simulink library "SUB_ECU_CruiseController"  (R2018a)
settings: Solver=VariableStepAuto  StartTime=0.0  StopTime=10.0  RelTol=1e-3
undefined symbols (not defined in the file or in its folder): ENUM_J1939_SWITCH_T
libraries: PTC_MBDS_LIB x17, simulink x4, simulink_extras x1
settings Model: Creator=Sundeep.Tuteja  LastModifiedBy=Sundeep.Tuteja

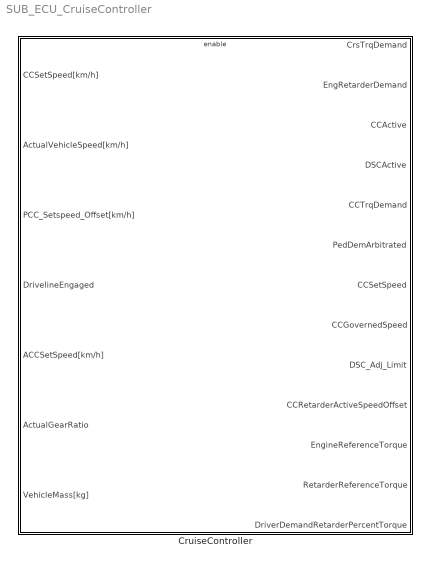
== system SUB_ECU_CruiseController ==
  CruiseController : Subsystem

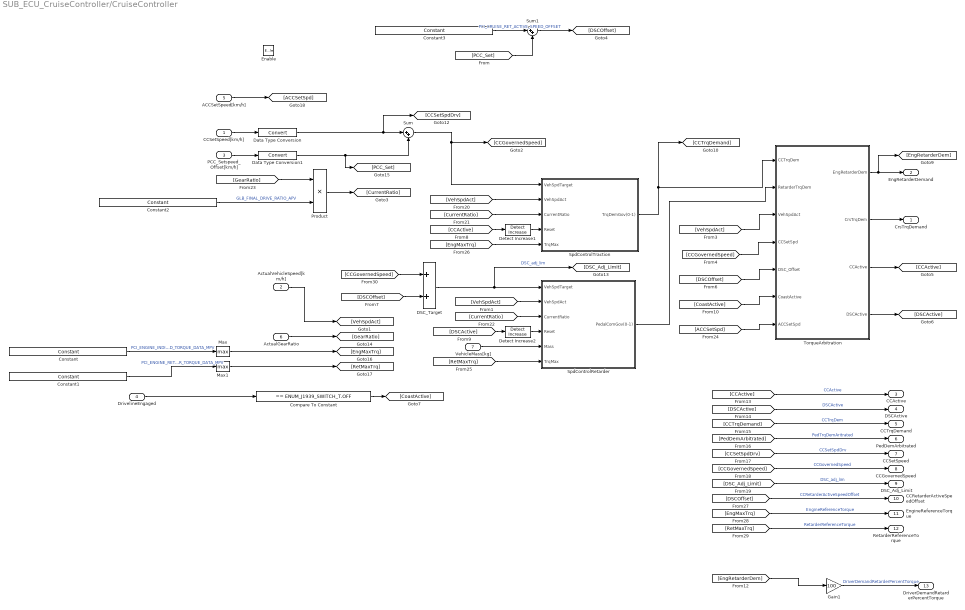
== system SUB_ECU_CruiseController/CruiseController ==
  CCSetSpeed[km/h] : Inport  Unit=km/h
  ActualVehicleSpeed[km/h] : Inport  Port=2  Unit=km/h
  PCC_Setspeed_Offset[km/h] : Inport  Port=3  Unit=km/h
  DrivelineEngaged : Inport  Port=4
  ACCSetSpeed[km/h] : Inport  Port=5  Unit=km/h
  ActualGearRatio : Inport  Port=6
  VehicleMass[kg] : Inport  Port=7  Unit=kg
  Enable : EnablePort
  Compare To Constant : simulink/Logic and Bit Operations/Compare To Constant  relop===  const=ENUM_J1939_SWITCH_T.OFF  OutDataTypeStr=boolean
  Constant : PTC_MBDS_LIB/Extras/Sources/Constant  Value2=PCI_ENGINE_INDICATED_TORQUE_DATA_MPV  PTC_MBDS_BlockVersion=5.41  PTC_BlockType=PTC_MBDS_Constant
      settings: SourceProductName=PACCAR Technical Center MBDS Library
      settings: AttributesFormatString=|
      | Value: <1 X 16>
      | Unit: 'N*m'
  Constant1 : PTC_MBDS_LIB/Extras/Sources/Constant  Value2=PCI_ENGINE_RETARDER_TORQUE_DATA_MPV  PTC_MBDS_BlockVersion=5.41  PTC_BlockType=PTC_MBDS_Constant
      settings: SourceProductName=PACCAR Technical Center MBDS Library
      settings: AttributesFormatString=|
      | Value: <1 X 16>
      | Unit: 'N*m'
  Constant2 : PTC_MBDS_LIB/Extras/Sources/Constant  Value2=GLB_FINAL_DRIVE_RATIO_APV  PTC_MBDS_BlockVersion=5.41  PTC_BlockType=PTC_MBDS_Constant
      settings: SourceProductName=PACCAR Technical Center MBDS Library
      settings: AttributesFormatString=|
      | Value: 2.64
      | Unit: '1'
  Constant3 : PTC_MBDS_LIB/Extras/Sources/Constant  Value2=PCI_CRUISE_RET_ACTIVE_SPEED_OFFSET  PTC_MBDS_BlockVersion=5.41  PTC_BlockType=PTC_MBDS_Constant
      settings: SourceProductName=PACCAR Technical Center MBDS Library
      settings: AttributesFormatString=|
      | Value: 4.5
      | Unit: 'km/h'
  DSC_Target : Sum
  Data Type Conversion : DataTypeConversion  SaturateOnIntegerOverflow=on
  Data Type Conversion1 : DataTypeConversion  SaturateOnIntegerOverflow=on
  Detect Increase1 : simulink/Logic and Bit Operations/Detect Increase  RequirementInfo={} %GIDa_b76eb822_ce3a_4747_9d7e_f46469754665  vinit=0.0  OutDataTypeStr=boolean
  Detect Increase2 : simulink/Logic and Bit Operations/Detect Increase  RequirementInfo={} %GIDa_136ab55b_ef96_43b5_a251_f5d87d11e975  vinit=0.0  OutDataTypeStr=boolean
  Gain1 : Gain  Gain=100
  Max : MinMax  Function=max  OutDataTypeStr=Inherit: Inherit via back propagation  SaturateOnIntegerOverflow=on  InputSameDT=on
  Max1 : MinMax  Function=max  OutDataTypeStr=Inherit: Inherit via back propagation  SaturateOnIntegerOverflow=on  InputSameDT=on
  Product : Product
  SpdControlRetarder : Subsystem
  SpdControlTraction : Subsystem
  Sum : Sum  Inputs=|++
  Sum1 : Sum  Inputs=|++
  TorqueArbitration : Subsystem
  CrsTrqDemand : Outport
  EngRetarderDemand : Outport  Port=2
  CCActive : Outport  Port=3
  DSCActive : Outport  Port=4
  CCTrqDemand : Outport  Port=5
  PedDemArbitrated : Outport  Port=6
  CCSetSpeed : Outport  Port=7
  CCGovernedSpeed : Outport  Port=8
  DSC_Adj_Limit : Outport  Port=9
  CCRetarderActiveSpeedOffset : Outport  Port=10
  EngineReferenceTorque : Outport  Port=11
  RetarderReferenceTorque : Outport  Port=12
  DriverDemandRetarderPercentTorque : Outport  Port=13
  wires:
  CCSetSpeed[km/h]/1 -> Data Type Conversion/1
  DSC_Target/1 -> [DSC_Adj_Limit], SpdControlRetarder/1(VehSpdTarget)  "DSC_adj_lim"
  Constant3/1 -> Sum1/1  "PCI_CRUISE_RET_ACTIVE_SPEED_OFFSET"
  SpdControlRetarder/1(PedalComGov(0-1)) -> TorqueArbitration/2(RetarderTrqDem)
  [VehSpdAct] -> SpdControlRetarder/2(VehSpdAct)
  [VehSpdAct] -> TorqueArbitration/3(VehSpdAct)
  [CCGovernedSpeed] -> DSC_Target/1
  [CCGovernedSpeed] -> TorqueArbitration/4(CCSetSpd)
  [DSCOffset] -> TorqueArbitration/5(DSC_Offset)
  [DSCOffset] -> DSC_Target/2
  TorqueArbitration/2(CrsTrqDem) -> CrsTrqDemand/1
  TorqueArbitration/1(EngRetarderDem) -> [EngRetarderDem], EngRetarderDemand/1
  TorqueArbitration/3(CCActive) -> [CCActive]
  TorqueArbitration/4(DSCActive) -> [DSCActive]
  Detect Increase1/1 -> SpdControlTraction/4(Reset)
  Detect Increase2/1 -> SpdControlRetarder/4(Reset)
  [CCActive] -> Detect Increase1/1
  [DSCActive] -> Detect Increase2/1
  DrivelineEngaged/1 -> Compare To Constant/1
  [CoastActive] -> TorqueArbitration/6(CoastActive)
  [CCActive] -> CCActive/1  "CCActive"
  [DSCActive] -> DSCActive/1  "DSCActive"
  SpdControlTraction/1(TrqDemGov(0-1)) -> TorqueArbitration/1(CCTrqDem), [CCTrqDemand]
  [CCTrqDemand] -> CCTrqDemand/1  "CCTrqDem"
  [PedDemArbitrated] -> PedDemArbitrated/1  "PedTrqDemAritrated"
  Sum/1 -> SpdControlTraction/1(VehSpdTarget), [CCGovernedSpeed]
  PCC_Setspeed_Offset[km/h]/1 -> Data Type Conversion1/1
  [CCSetSpdDrv] -> CCSetSpeed/1  "CCSetSpdDrv"
  [CCGovernedSpeed] -> CCGovernedSpeed/1  "CCGovernedSpeed"
  [DSC_Adj_Limit] -> DSC_Adj_Limit/1  "DSC_adj_lim"
  Constant2/1 -> Product/2  "GLB_FINAL_DRIVE_RATIO_APV"
  ActualVehicleSpeed[km/h]/1 -> [VehSpdAct]
  Product/1 -> [CurrentRatio]
  [VehSpdAct] -> SpdControlTraction/2(VehSpdAct)
  [CurrentRatio] -> SpdControlTraction/3(CurrentRatio)
  [CurrentRatio] -> SpdControlRetarder/3(CurrentRatio)
  VehicleMass[kg]/1 -> SpdControlRetarder/5(Mass)
  ActualGearRatio/1 -> [GearRatio]
  [GearRatio] -> Product/1
  Constant/1 -> Max/1  "PCI_ENGINE_INDICATED_TORQUE_DATA_MPV"
  Max1/1 -> [RetMaxTrq]
  [RetMaxTrq] -> SpdControlRetarder/6(TrqMax)
  [EngMaxTrq] -> SpdControlTraction/5(TrqMax)
  ACCSetSpeed[km/h]/1 -> [ACCSetSpd]
  [ACCSetSpd] -> TorqueArbitration/7(ACCSetSpd)
  Sum1/1 -> [DSCOffset]
  [PCC_Set] -> Sum1/2
  Max/1 -> [EngMaxTrq]
  Constant1/1 -> Max1/1  "PCI_ENGINE_RETARDER_TORQUE_DATA_MPV"
  Compare To Constant/1 -> [CoastActive]
  [DSCOffset] -> CCRetarderActiveSpeedOffset/1  "CCRetarderActiveSpeedOffset"
  [EngMaxTrq] -> EngineReferenceTorque/1  "EngineReferenceTorque"
  [RetMaxTrq] -> RetarderReferenceTorque/1  "RetarderReferenceTorque"
  Data Type Conversion/1 -> [CCSetSpdDrv], Sum/1
  Data Type Conversion1/1 -> [PCC_Set], Sum/2
  Gain1/1 -> DriverDemandRetarderPercentTorque/1  "DriverDemandRetarderPercentTorque"
  [EngRetarderDem] -> Gain1/1

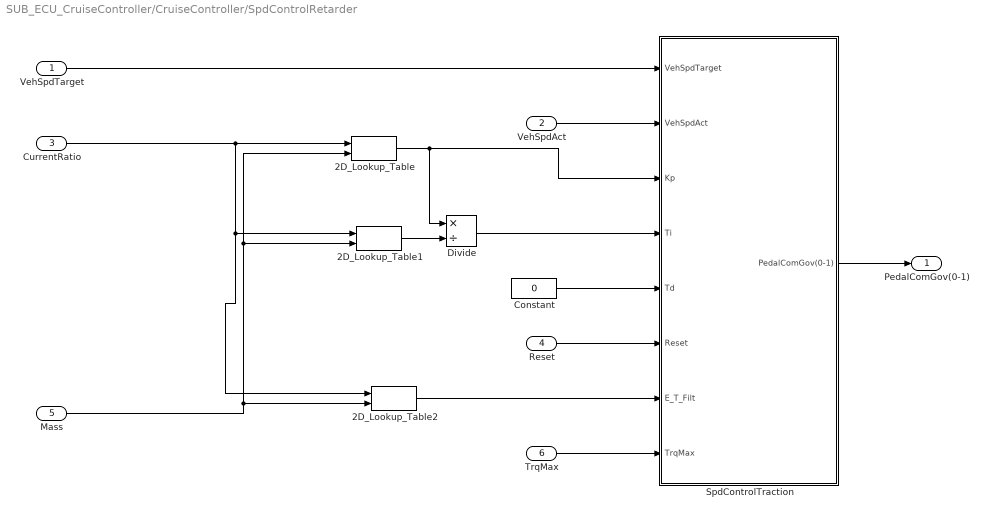
== system SUB_ECU_CruiseController/CruiseController/SpdControlRetarder ==
  VehSpdTarget : Inport
  VehSpdAct : Inport  Port=2
  CurrentRatio : Inport  Port=3
  Reset : Inport  Port=4
  Mass : Inport  Port=5
  TrqMax : Inport  Port=6
  2D_Lookup_Table : PTC_MBDS_LIB/Extras/Lookup Tables/2D_Lookup_Table  ParameterObjectName=PCI_CRUISE_DSC_KP_DATA_MPV  PTC_MBDS_BlockVersion=5.41  PTC_BlockType=PTC_MBDS_2D_Lookup_Table
      settings: SourceProductName=PACCAR Technical Center MBDS Library
      settings: AttributesFormatString=|
      | Row Axis: PCI_CRUISE_DSC_DRIVE_RATIO_MPV ()
      | Column Axis: PCI_CRUISE_DSC_MASS_MPV (kg)
      | Data Axis: PCI_CRUISE_DSC_KP_DATA_MPV ()
  2D_Lookup_Table1 : PTC_MBDS_LIB/Extras/Lookup Tables/2D_Lookup_Table  ParameterObjectName=PCI_CRUISE_DSC_KI_DATA_MPV  PTC_MBDS_BlockVersion=5.41  PTC_BlockType=PTC_MBDS_2D_Lookup_Table
      settings: SourceProductName=PACCAR Technical Center MBDS Library
      settings: AttributesFormatString=|
      | Row Axis: PCI_CRUISE_DSC_DRIVE_RATIO_MPV ()
      | Column Axis: PCI_CRUISE_DSC_MASS_MPV (kg)
      | Data Axis: PCI_CRUISE_DSC_KI_DATA_MPV (1/s)
  2D_Lookup_Table2 : PTC_MBDS_LIB/Extras/Lookup Tables/2D_Lookup_Table  ParameterObjectName=PCI_CRUISE_DSC_ERROR_FILT_T_MPV  PTC_MBDS_BlockVersion=5.41  PTC_BlockType=PTC_MBDS_2D_Lookup_Table
      settings: SourceProductName=PACCAR Technical Center MBDS Library
      settings: AttributesFormatString=|
      | Row Axis: PCI_CRUISE_DSC_DRIVE_RATIO_MPV ()
      | Column Axis: PCI_CRUISE_DSC_MASS_MPV (kg)
      | Data Axis: PCI_CRUISE_DSC_ERROR_FILT_T_MPV (s)
  Constant : Constant  Value=0
  Divide : Product  Inputs=*/
  SpdControlTraction : Subsystem
  PedalComGov(0-1) : Outport
  wires:
  Mass/1 -> 2D_Lookup_Table2/2, 2D_Lookup_Table1/2, 2D_Lookup_Table/2
  VehSpdTarget/1 -> SpdControlTraction/1(VehSpdTarget)
  VehSpdAct/1 -> SpdControlTraction/2(VehSpdAct)
  SpdControlTraction/1(PedalComGov(0-1)) -> PedalComGov(0-1)/1
  Reset/1 -> SpdControlTraction/6(Reset)
  CurrentRatio/1 -> 2D_Lookup_Table/1, 2D_Lookup_Table2/1, 2D_Lookup_Table1/1
  2D_Lookup_Table2/1 -> SpdControlTraction/7(E_T_Filt)
  Constant/1 -> SpdControlTraction/5(Td)
  2D_Lookup_Table/1 -> SpdControlTraction/3(Kp), Divide/1
  2D_Lookup_Table1/1 -> Divide/2
  Divide/1 -> SpdControlTraction/4(Ti)
  TrqMax/1 -> SpdControlTraction/8(TrqMax)

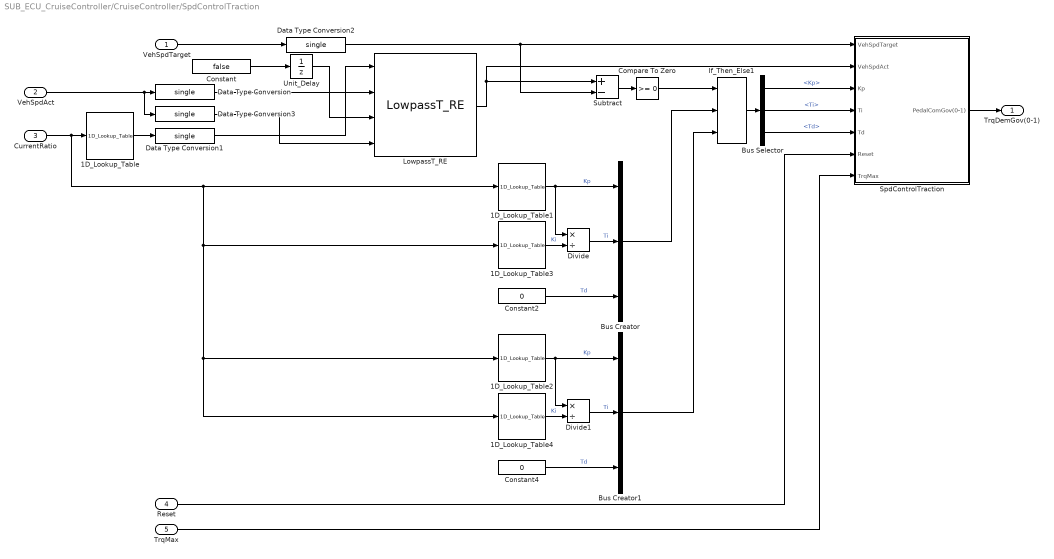
== system SUB_ECU_CruiseController/CruiseController/SpdControlTraction ==
  VehSpdTarget : Inport
  VehSpdAct : Inport  Port=2
  CurrentRatio : Inport  Port=3
  Reset : Inport  Port=4
  TrqMax : Inport  Port=5
  1D_Lookup_Table : PTC_MBDS_LIB/Extras/Lookup Tables/1D_Lookup_Table  ParameterObjectName=PCI_VSPD_FILT_T_DATA_MPV  PTC_MBDS_BlockVersion=5.41  PTC_BlockType=PTC_MBDS_1D_Lookup_Table
      settings: SourceProductName=PACCAR Technical Center MBDS Library
      settings: AttributesFormatString=|
      | X Axis: PCI_DRIVE_RATIO_MPV (1)
      | Y Axis: PCI_VSPD_FILT_T_DATA_MPV (s)
  1D_Lookup_Table1 : PTC_MBDS_LIB/Extras/Lookup Tables/1D_Lookup_Table  ParameterObjectName=PCI_CRUISE_KP_HIGH_MPV  PTC_MBDS_BlockVersion=5.41  PTC_BlockType=PTC_MBDS_1D_Lookup_Table
      settings: SourceProductName=PACCAR Technical Center MBDS Library
      settings: AttributesFormatString=|
      | X Axis: PCI_DRIVE_RATIO_MPV (1)
      | Y Axis: PCI_CRUISE_KP_HIGH_MPV (1)
  1D_Lookup_Table2 : PTC_MBDS_LIB/Extras/Lookup Tables/1D_Lookup_Table  ParameterObjectName=PCI_CRUISE_KP_LOW_MPV  PTC_MBDS_BlockVersion=5.41  PTC_BlockType=PTC_MBDS_1D_Lookup_Table
      settings: SourceProductName=PACCAR Technical Center MBDS Library
      settings: AttributesFormatString=|
      | X Axis: PCI_DRIVE_RATIO_MPV (1)
      | Y Axis: PCI_CRUISE_KP_LOW_MPV ()
  1D_Lookup_Table3 : PTC_MBDS_LIB/Extras/Lookup Tables/1D_Lookup_Table  ParameterObjectName=PCI_CRUISE_KI_HIGH_MPV  PTC_MBDS_BlockVersion=5.41  PTC_BlockType=PTC_MBDS_1D_Lookup_Table
      settings: SourceProductName=PACCAR Technical Center MBDS Library
      settings: AttributesFormatString=|
      | X Axis: PCI_DRIVE_RATIO_MPV (1)
      | Y Axis: PCI_CRUISE_KI_HIGH_MPV (1/s)
  1D_Lookup_Table4 : PTC_MBDS_LIB/Extras/Lookup Tables/1D_Lookup_Table  ParameterObjectName=PCI_CRUISE_KI_LOW_MPV  PTC_MBDS_BlockVersion=5.41  PTC_BlockType=PTC_MBDS_1D_Lookup_Table
      settings: SourceProductName=PACCAR Technical Center MBDS Library
      settings: AttributesFormatString=|
      | X Axis: PCI_DRIVE_RATIO_MPV (1)
      | Y Axis: PCI_CRUISE_KI_LOW_MPV (1/s)
  Bus Creator : BusCreator  Inputs=3
  Bus Creator1 : BusCreator  Inputs=3
  Bus Selector : BusSelector  OutputSignals=Kp,Ti,Td
  Compare To Zero : simulink/Logic and Bit Operations/Compare To Zero  relop=>=  OutDataTypeStr=boolean
  Constant : Constant  Value=false  OutDataTypeStr=boolean
  Constant2 : Constant  Value=0
  Constant4 : Constant  Value=0
  Data Type Conversion{,1..3} (4 alike) : DataTypeConversion  OutDataTypeStr=single
  Divide : Product  Inputs=*/
  Divide1 : Product  Inputs=*/
  If_Then_Else1 : PTC_MBDS_LIB/Extras/Signal Routing/If_Then_Else  PTC_MBDS_BlockVersion=5.41  PTC_BlockType=PTC_MBDS_If_Then_Else
      settings: SourceProductName=PACCAR Technical Center MBDS Library
  LowpassT_RE : PTC_MBDS_LIB/MBDS Standard Library/Extended Operations/Filters/LowpassT_RE  dT_Enabled=off  dT=GLB_FIXED_STEP_SIZE_CPV  E_Enabled=off  R_Enabled=on  IV_Enabled=on  IV=0  PTC_MBDS_BlockVersion=5.41  PTC_BlockType=PTC_MBDS_LowpassT_RE
      settings: AttributesFormatString=dT = %<dT>  SourceProductName=PACCAR Technical Center MBDS Library
  SpdControlTraction : Subsystem
  Subtract : Sum  Inputs=+-
  Unit_Delay : UnitDelay  InitialCondition=true  SampleTime=-1
      settings: AttributesFormatString=Init = %<InitialCondition>
  TrqDemGov(0-1) : Outport
  wires:
  Reset/1 -> SpdControlTraction/6(Reset)
  SpdControlTraction/1(PedalComGov(0-1)) -> TrqDemGov(0-1)/1
  VehSpdTarget/1 -> Data Type Conversion2/1
  CurrentRatio/1 -> 1D_Lookup_Table/1, 1D_Lookup_Table1/1, 1D_Lookup_Table3/1, 1D_Lookup_Table4/1, 1D_Lookup_Table2/1
  VehSpdAct/1 -> Data Type Conversion3/1, Data Type Conversion/1
  Constant/1 -> Unit_Delay/1
  1D_Lookup_Table3/1 -> Divide/2  "Ki"
  1D_Lookup_Table1/1 -> Divide/1, Bus Creator/1  "Kp"
  Divide/1 -> Bus Creator/2  "Ti"
  Constant2/1 -> Bus Creator/3  "Td"
  1D_Lookup_Table4/1 -> Divide1/2  "Ki"
  1D_Lookup_Table2/1 -> Divide1/1, Bus Creator1/1  "Kp"
  Divide1/1 -> Bus Creator1/2  "Ti"
  Constant4/1 -> Bus Creator1/3  "Td"
  Bus Creator/1 -> If_Then_Else1/2
  Bus Creator1/1 -> If_Then_Else1/3
  LowpassT_RE/1 -> SpdControlTraction/2(VehSpdAct), Subtract/1
  Subtract/1 -> Compare To Zero/1
  Compare To Zero/1 -> If_Then_Else1/1
  If_Then_Else1/1 -> Bus Selector/1
  Bus Selector/1 -> SpdControlTraction/3(Kp)  "<Kp>"
  Bus Selector/2 -> SpdControlTraction/4(Ti)  "<Ti>"
  Bus Selector/3 -> SpdControlTraction/5(Td)  "<Td>"
  1D_Lookup_Table/1 -> Data Type Conversion1/1
  Data Type Conversion2/1 -> Subtract/2, SpdControlTraction/1(VehSpdTarget)
  TrqMax/1 -> SpdControlTraction/7(TrqMax)
  Data Type Conversion1/1 -> LowpassT_RE/1
  Data Type Conversion/1 -> LowpassT_RE/2
  Data Type Conversion3/1 -> LowpassT_RE/4
  Unit_Delay/1 -> LowpassT_RE/3

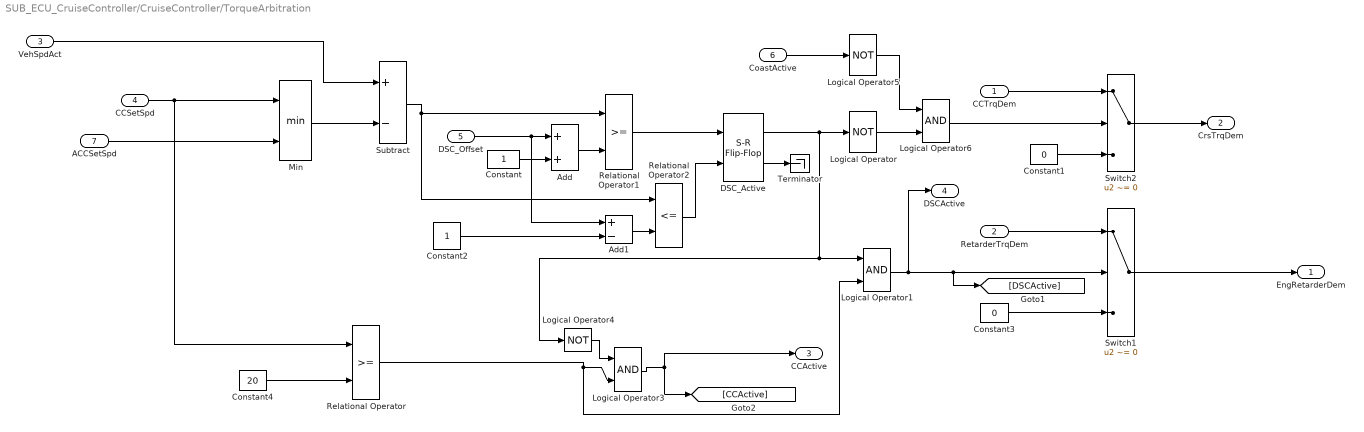
== system SUB_ECU_CruiseController/CruiseController/TorqueArbitration ==
  CCTrqDem : Inport
  RetarderTrqDem : Inport  Port=2
  VehSpdAct : Inport  Port=3
  CCSetSpd : Inport  Port=4
  DSC_Offset : Inport  Port=5
  CoastActive : Inport  Port=6
  ACCSetSpd : Inport  Port=7
  Add : Sum
  Add1 : Sum  Inputs=+-
  Constant : Constant
  Constant1 : Constant  Value=0
  Constant2 : Constant
  Constant3 : Constant  Value=0
  Constant4 : Constant  Value=20
  DSC_Active : simulink_extras/Flip Flops/S-R Flip-Flop  RequirementInfo={} %GIDa_1255c0f1_5c67_4298_b231_ebbb996d878f  initial_condition=0
  Logical Operator : Logic  Operator=NOT  AllPortsSameDT=off  OutDataTypeStr=boolean
  Logical Operator1 : Logic  AllPortsSameDT=off  OutDataTypeStr=boolean
  Logical Operator3 : Logic  AllPortsSameDT=off  OutDataTypeStr=boolean
  Logical Operator4 : Logic  Operator=NOT  AllPortsSameDT=off  OutDataTypeStr=boolean
  Logical Operator5 : Logic  Operator=NOT  AllPortsSameDT=off  OutDataTypeStr=boolean
  Logical Operator6 : Logic  AllPortsSameDT=off  OutDataTypeStr=boolean
  Min : MinMax  Inputs=2  OutDataTypeStr=Inherit: Inherit via back propagation  SaturateOnIntegerOverflow=on  InputSameDT=on
  Relational Operator : RelationalOperator  OutDataTypeStr=boolean  RndMeth=Nearest
  Relational Operator1 : RelationalOperator  OutDataTypeStr=boolean  RndMeth=Nearest
  Relational Operator2 : RelationalOperator  Operator=<=  OutDataTypeStr=boolean  RndMeth=Nearest
  Subtract : Sum  Inputs=+-
  Switch1 : Switch  Criteria=u2 ~= 0
  Switch2 : Switch  Criteria=u2 ~= 0
  Terminator : Terminator
  EngRetarderDem : Outport
  CrsTrqDem : Outport  Port=2
  CCActive : Outport  Port=3
  DSCActive : Outport  Port=4
  wires:
  Logical Operator3/1 -> CCActive/1, [CCActive]
  Relational Operator2/1 -> DSC_Active/2
  Constant4/1 -> Relational Operator/2
  Relational Operator1/1 -> DSC_Active/1
  Constant/1 -> Add/2
  Subtract/1 -> Relational Operator2/1, Relational Operator1/1
  VehSpdAct/1 -> Subtract/1
  Switch1/1 -> EngRetarderDem/1
  Switch2/1 -> CrsTrqDem/1
  RetarderTrqDem/1 -> Switch1/1
  Constant3/1 -> Switch1/3
  Constant1/1 -> Switch2/3
  DSC_Offset/1 -> Add/1, Add1/1
  Add/1 -> Relational Operator1/2
  CCTrqDem/1 -> Switch2/1
  Logical Operator/1 -> Logical Operator6/2
  DSC_Active/1 -> Logical Operator/1, Logical Operator1/1, Logical Operator4/1
  Logical Operator1/1 -> [DSCActive], Switch1/2, DSCActive/1
  Relational Operator/1 -> Logical Operator1/2, Logical Operator3/2
  Logical Operator4/1 -> Logical Operator3/1
  CoastActive/1 -> Logical Operator5/1
  Logical Operator6/1 -> Switch2/2
  Logical Operator5/1 -> Logical Operator6/1
  DSC_Active/2 -> Terminator/1
  Add1/1 -> Relational Operator2/2
  Constant2/1 -> Add1/2
  Min/1 -> Subtract/2
  CCSetSpd/1 -> Relational Operator/1, Min/1
  ACCSetSpd/1 -> Min/2

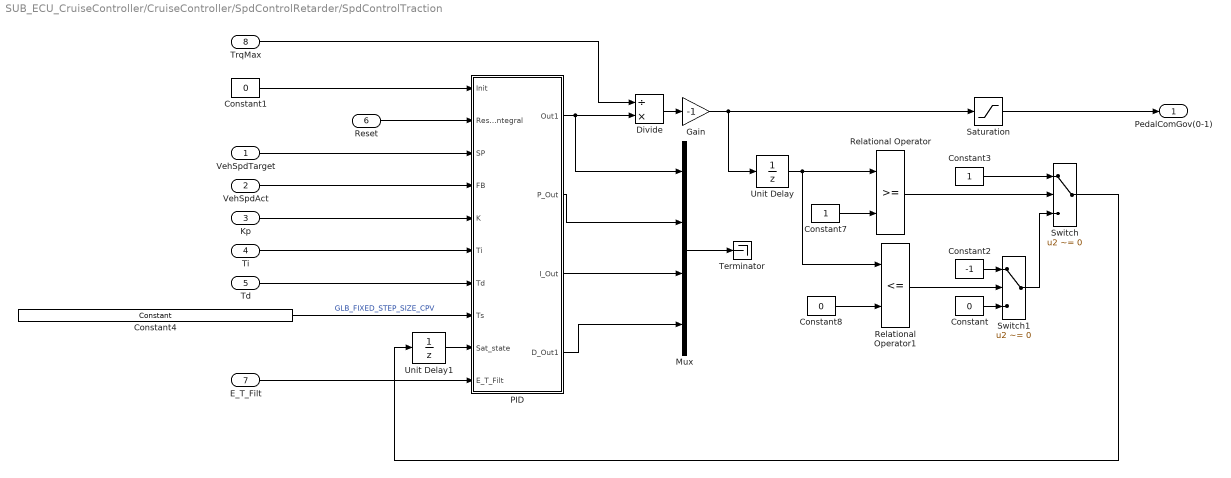
== system SUB_ECU_CruiseController/CruiseController/SpdControlRetarder/SpdControlTraction ==
  VehSpdTarget : Inport
  VehSpdAct : Inport  Port=2
  Kp : Inport  Port=3
  Ti : Inport  Port=4
  Td : Inport  Port=5
  Reset : Inport  Port=6
  E_T_Filt : Inport  Port=7
  TrqMax : Inport  Port=8
  Constant : Constant  Value=0
  Constant1 : Constant  Value=0
  Constant2 : Constant  Value=-1
  Constant3 : Constant
  Constant4 : PTC_MBDS_LIB/Extras/Sources/Constant  Value2=GLB_FIXED_STEP_SIZE_CPV  PTC_MBDS_BlockVersion=5.41  PTC_BlockType=PTC_MBDS_Constant
      settings: SourceProductName=PACCAR Technical Center MBDS Library
      settings: AttributesFormatString=|
      | Value: 0.01
      | Unit: 's'
  Constant7 : Constant
  Constant8 : Constant  Value=0
  Divide : Product  Inputs=/*
  Gain : Gain  Gain=-1
  Mux : Mux
  PID : Subsystem
  Relational Operator : RelationalOperator  OutDataTypeStr=boolean  RndMeth=Nearest
  Relational Operator1 : RelationalOperator  Operator=<=  OutDataTypeStr=boolean  RndMeth=Nearest
  Saturation : Saturate  UpperLimit=1  LowerLimit=0
  Switch : Switch  Criteria=u2 ~= 0
  Switch1 : Switch  Criteria=u2 ~= 0
  Terminator : Terminator
  Unit Delay : UnitDelay  SampleTime=-1
  Unit Delay1 : UnitDelay  SampleTime=-1
  PedalComGov(0-1) : Outport
  wires:
  Saturation/1 -> PedalComGov(0-1)/1
  PID/1(Out1) -> Mux/1, Divide/2
  VehSpdAct/1 -> PID/4(FB)
  VehSpdTarget/1 -> PID/3(SP)
  Constant4/1 -> PID/8(Ts)  "GLB_FIXED_STEP_SIZE_CPV"
  Td/1 -> PID/7(Td)
  Ti/1 -> PID/6(Ti)
  Kp/1 -> PID/5(K)
  Constant1/1 -> PID/1(Init)
  Mux/1 -> Terminator/1
  PID/2(P_Out) -> Mux/2
  PID/3(I_Out) -> Mux/3
  PID/4(D_Out1) -> Mux/4
  Relational Operator1/1 -> Switch1/2
  Constant/1 -> Switch1/3
  Constant2/1 -> Switch1/1
  Switch1/1 -> Switch/3
  Constant3/1 -> Switch/1
  Switch/1 -> Unit Delay1/1
  Relational Operator/1 -> Switch/2
  Constant7/1 -> Relational Operator/2
  Constant8/1 -> Relational Operator1/2
  Unit Delay/1 -> Relational Operator/1, Relational Operator1/1
  Reset/1 -> PID/2(Reset_Integral)
  Unit Delay1/1 -> PID/9(Sat_state)
  Gain/1 -> Saturation/1, Unit Delay/1
  E_T_Filt/1 -> PID/10(E_T_Filt)
  Divide/1 -> Gain/1
  TrqMax/1 -> Divide/1

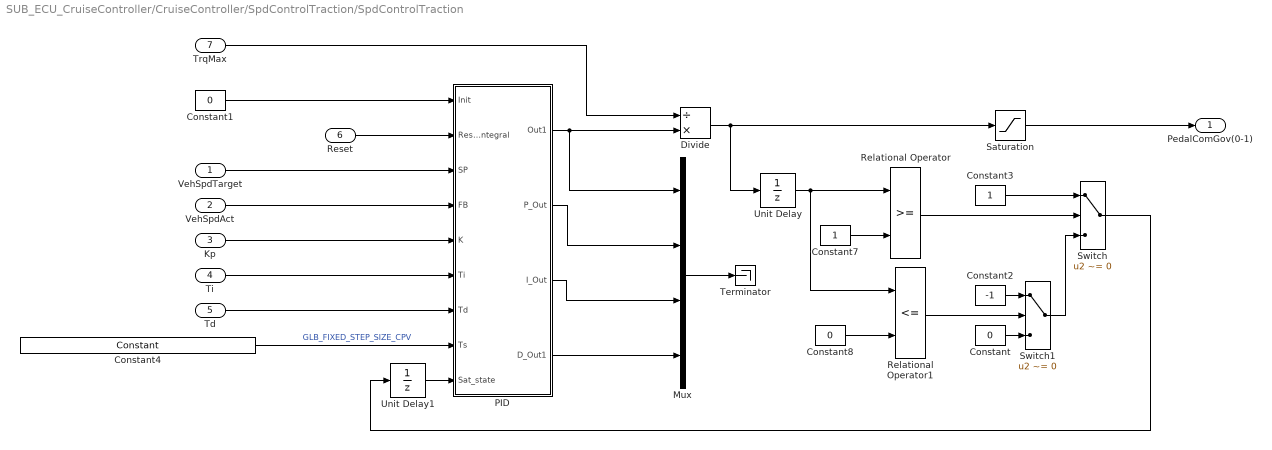
== system SUB_ECU_CruiseController/CruiseController/SpdControlTraction/SpdControlTraction ==
  VehSpdTarget : Inport
  VehSpdAct : Inport  Port=2
  Kp : Inport  Port=3
  Ti : Inport  Port=4
  Td : Inport  Port=5
  Reset : Inport  Port=6
  TrqMax : Inport  Port=7
  Constant : Constant  Value=0
  Constant1 : Constant  Value=0
  Constant2 : Constant  Value=-1
  Constant3 : Constant
  Constant4 : PTC_MBDS_LIB/Extras/Sources/Constant  Value2=GLB_FIXED_STEP_SIZE_CPV  PTC_MBDS_BlockVersion=5.41  PTC_BlockType=PTC_MBDS_Constant
      settings: SourceProductName=PACCAR Technical Center MBDS Library
      settings: AttributesFormatString=|
      | Value: 0.01
      | Unit: 's'
  Constant7 : Constant
  Constant8 : Constant  Value=0
  Divide : Product  Inputs=/*
  Mux : Mux
  PID : Subsystem
  Relational Operator : RelationalOperator  OutDataTypeStr=boolean  RndMeth=Nearest
  Relational Operator1 : RelationalOperator  Operator=<=  OutDataTypeStr=boolean  RndMeth=Nearest
  Saturation : Saturate  UpperLimit=1  LowerLimit=0
  Switch : Switch  Criteria=u2 ~= 0
  Switch1 : Switch  Criteria=u2 ~= 0
  Terminator : Terminator
  Unit Delay : UnitDelay  SampleTime=-1
  Unit Delay1 : UnitDelay  SampleTime=-1
  PedalComGov(0-1) : Outport
  wires:
  Unit Delay1/1 -> PID/9(Sat_state)
  Reset/1 -> PID/2(Reset_Integral)
  Unit Delay/1 -> Relational Operator1/1, Relational Operator/1
  Constant8/1 -> Relational Operator1/2
  Constant7/1 -> Relational Operator/2
  Relational Operator/1 -> Switch/2
  Switch/1 -> Unit Delay1/1
  Constant3/1 -> Switch/1
  Switch1/1 -> Switch/3
  Constant2/1 -> Switch1/1
  Constant/1 -> Switch1/3
  Relational Operator1/1 -> Switch1/2
  PID/4(D_Out1) -> Mux/4
  PID/3(I_Out) -> Mux/3
  PID/2(P_Out) -> Mux/2
  Mux/1 -> Terminator/1
  Constant1/1 -> PID/1(Init)
  Kp/1 -> PID/5(K)
  Ti/1 -> PID/6(Ti)
  Td/1 -> PID/7(Td)
  Constant4/1 -> PID/8(Ts)  "GLB_FIXED_STEP_SIZE_CPV"
  VehSpdTarget/1 -> PID/3(SP)
  VehSpdAct/1 -> PID/4(FB)
  Divide/1 -> Unit Delay/1, Saturation/1
  Saturation/1 -> PedalComGov(0-1)/1
  PID/1(Out1) -> Divide/2, Mux/1
  TrqMax/1 -> Divide/1

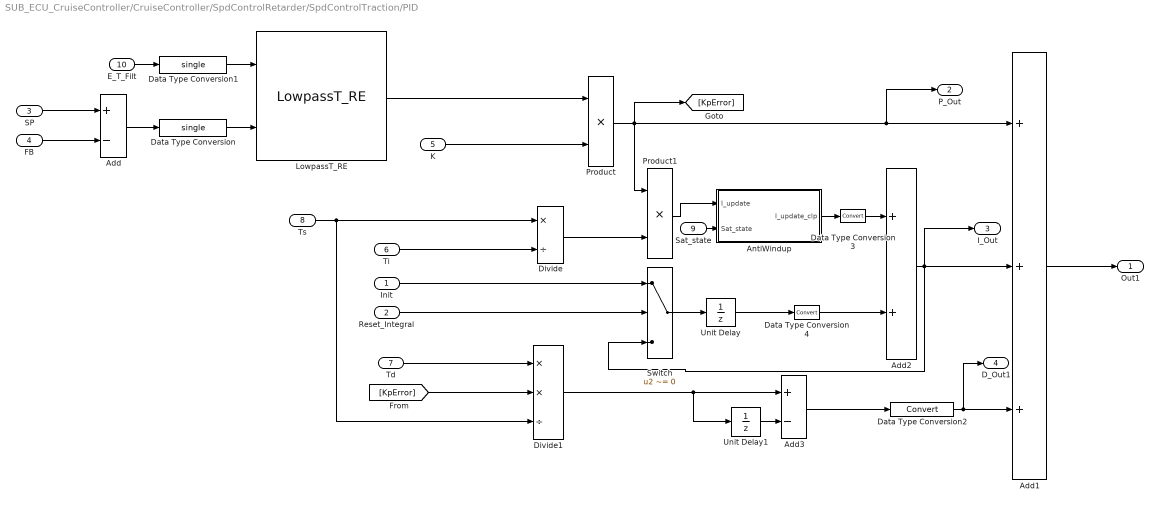
== system SUB_ECU_CruiseController/CruiseController/SpdControlRetarder/SpdControlTraction/PID ==
  Init : Inport
  Reset_Integral : Inport  Port=2
  SP : Inport  Port=3
  FB : Inport  Port=4
  K : Inport  Port=5
  Ti : Inport  Port=6
  Td : Inport  Port=7
  Ts : Inport  Port=8
  Sat_state : Inport  Port=9
  E_T_Filt : Inport  Port=10
  Add : Sum  Inputs=+-
  Add1 : Sum  Inputs=+++
  Add2 : Sum
  Add3 : Sum  Inputs=+-
  AntiWindup : Subsystem
  Data Type Conversion2 : DataTypeConversion  SaturateOnIntegerOverflow=on
  Data Type Conversion3 : DataTypeConversion  SaturateOnIntegerOverflow=on
  Data Type Conversion4 : DataTypeConversion  SaturateOnIntegerOverflow=on
  Data Type Conversion : DataTypeConversion  OutDataTypeStr=single
  Data Type Conversion1 : DataTypeConversion  OutDataTypeStr=single
  Divide : Product  Inputs=*/
  Divide1 : Product  Inputs=**/
  LowpassT_RE : PTC_MBDS_LIB/MBDS Standard Library/Extended Operations/Filters/LowpassT_RE  dT_Enabled=off  dT=GLB_FIXED_STEP_SIZE_CPV  E_Enabled=off  R_Enabled=off  IV_Enabled=off  IV=0  PTC_MBDS_BlockVersion=5.41  PTC_BlockType=PTC_MBDS_LowpassT_RE
      settings: SourceProductName=PACCAR Technical Center MBDS Library
      settings: AttributesFormatString=|
      | IV = %<IV>
      | dT = %<dT>
  Product : Product  RndMeth=Zero
  Product1 : Product  RndMeth=Zero
  Switch : Switch  Criteria=u2 ~= 0
  Unit Delay : UnitDelay  SampleTime=-1
  Unit Delay1 : UnitDelay  SampleTime=-1
  Out1 : Outport
  P_Out : Outport  Port=2
  I_Out : Outport  Port=3
  D_Out1 : Outport  Port=4
  wires:
  Add3/1 -> Data Type Conversion2/1
  Unit Delay1/1 -> Add3/2
  Divide1/1 -> Unit Delay1/1, Add3/1
  [KpError] -> Divide1/2
  Td/1 -> Divide1/1
  Add1/1 -> Out1/1
  Add2/1 -> I_Out/1, Add1/2, Switch/3
  Switch/1 -> Unit Delay/1
  Unit Delay/1 -> Data Type Conversion4/1
  Divide/1 -> Product1/2
  Ti/1 -> Divide/2
  Ts/1 -> Divide/1, Divide1/3
  Product/1 -> P_Out/1, Add1/1, [KpError], Product1/1
  K/1 -> Product/2
  FB/1 -> Add/2
  SP/1 -> Add/1
  Init/1 -> Switch/1
  Reset_Integral/1 -> Switch/2
  AntiWindup/1(I_update_clp) -> Data Type Conversion3/1
  Product1/1 -> AntiWindup/1(I_update)
  Sat_state/1 -> AntiWindup/2(Sat_state)
  Add/1 -> Data Type Conversion/1
  E_T_Filt/1 -> Data Type Conversion1/1
  LowpassT_RE/1 -> Product/1
  Data Type Conversion/1 -> LowpassT_RE/2
  Data Type Conversion1/1 -> LowpassT_RE/1
  Data Type Conversion2/1 -> D_Out1/1, Add1/3
  Data Type Conversion3/1 -> Add2/1
  Data Type Conversion4/1 -> Add2/2

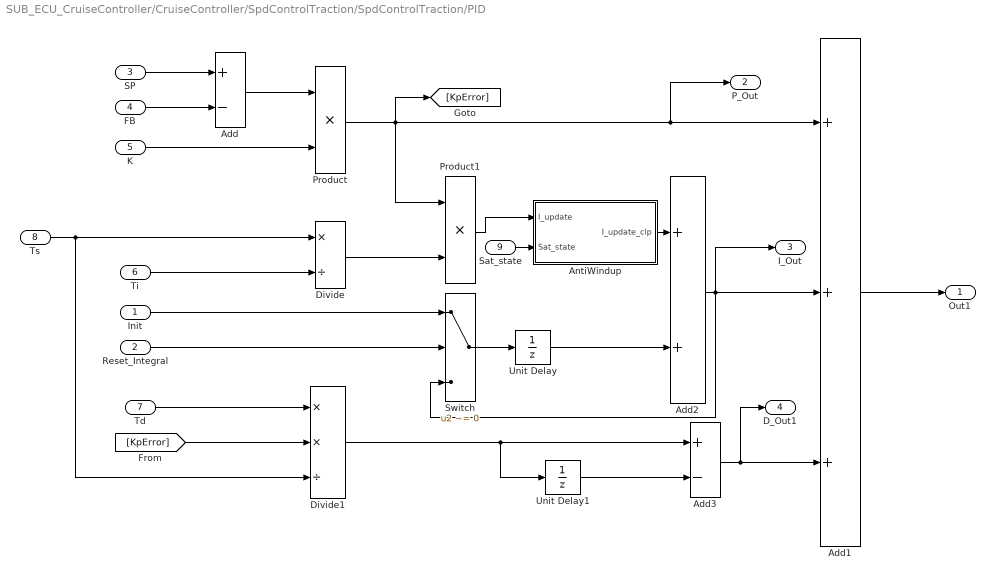
== system SUB_ECU_CruiseController/CruiseController/SpdControlTraction/SpdControlTraction/PID ==
  Init : Inport
  Reset_Integral : Inport  Port=2
  SP : Inport  Port=3
  FB : Inport  Port=4
  K : Inport  Port=5
  Ti : Inport  Port=6
  Td : Inport  Port=7
  Ts : Inport  Port=8
  Sat_state : Inport  Port=9
  Add : Sum  Inputs=+-
  Add1 : Sum  Inputs=+++
  Add2 : Sum
  Add3 : Sum  Inputs=+-
  AntiWindup : Subsystem
  Divide : Product  Inputs=*/
  Divide1 : Product  Inputs=**/
  Product : Product  RndMeth=Zero
  Product1 : Product  RndMeth=Zero
  Switch : Switch  Criteria=u2 ~= 0
  Unit Delay : UnitDelay  SampleTime=-1
  Unit Delay1 : UnitDelay  SampleTime=-1
  Out1 : Outport
  P_Out : Outport  Port=2
  I_Out : Outport  Port=3
  D_Out1 : Outport  Port=4
  wires:
  Sat_state/1 -> AntiWindup/2(Sat_state)
  Product1/1 -> AntiWindup/1(I_update)
  AntiWindup/1(I_update_clp) -> Add2/1
  Reset_Integral/1 -> Switch/2
  Init/1 -> Switch/1
  SP/1 -> Add/1
  FB/1 -> Add/2
  Add/1 -> Product/1
  K/1 -> Product/2
  Product/1 -> Product1/1, Add1/1, P_Out/1, [KpError]
  Ts/1 -> Divide1/3, Divide/1
  Ti/1 -> Divide/2
  Divide/1 -> Product1/2
  Unit Delay/1 -> Add2/2
  Switch/1 -> Unit Delay/1
  Add2/1 -> Switch/3, Add1/2, I_Out/1
  Add1/1 -> Out1/1
  Td/1 -> Divide1/1
  [KpError] -> Divide1/2
  Divide1/1 -> Add3/1, Unit Delay1/1
  Unit Delay1/1 -> Add3/2
  Add3/1 -> Add1/3, D_Out1/1

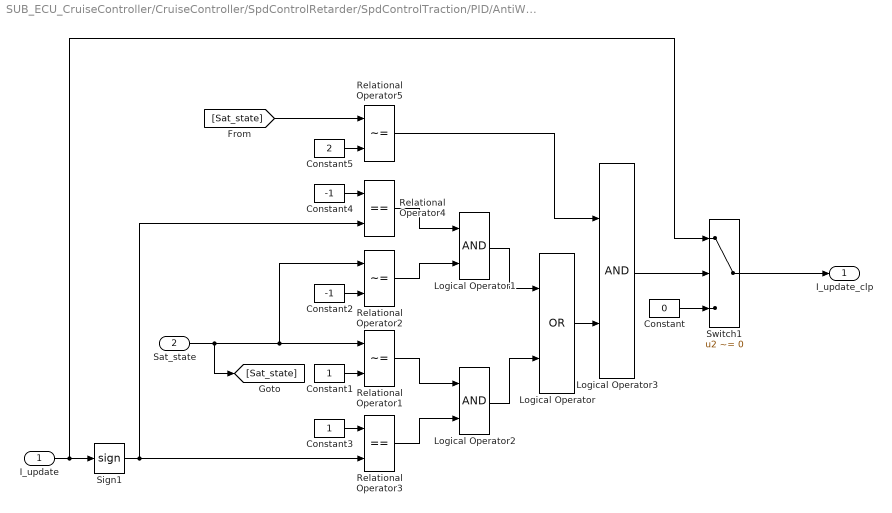
== system SUB_ECU_CruiseController/CruiseController/SpdControlRetarder/SpdControlTraction/PID/AntiWindup ==
  I_update : Inport
  Sat_state : Inport  Port=2
  Constant : Constant  Value=0
  Constant1 : Constant
  Constant2 : Constant  Value=-1
  Constant3 : Constant
  Constant4 : Constant  Value=-1
  Constant5 : Constant  Value=2
  Logical Operator : Logic  Operator=OR  AllPortsSameDT=off  OutDataTypeStr=boolean
  Logical Operator1 : Logic  AllPortsSameDT=off  OutDataTypeStr=boolean
  Logical Operator2 : Logic  AllPortsSameDT=off  OutDataTypeStr=boolean
  Logical Operator3 : Logic  AllPortsSameDT=off  OutDataTypeStr=boolean
  Relational Operator1 : RelationalOperator  Operator=~=  OutDataTypeStr=boolean  RndMeth=Nearest
  Relational Operator2 : RelationalOperator  Operator=~=  OutDataTypeStr=boolean  RndMeth=Nearest
  Relational Operator3 : RelationalOperator  Operator===  OutDataTypeStr=boolean  RndMeth=Nearest
  Relational Operator4 : RelationalOperator  Operator===  OutDataTypeStr=boolean  RndMeth=Nearest
  Relational Operator5 : RelationalOperator  Operator=~=  OutDataTypeStr=boolean  RndMeth=Nearest
  Sign1 : Signum
  Switch1 : Switch  Criteria=u2 ~= 0
  I_update_clp : Outport
  wires:
  Switch1/1 -> I_update_clp/1
  I_update/1 -> Sign1/1, Switch1/1
  Constant1/1 -> Relational Operator1/2
  Sat_state/1 -> Relational Operator1/1, Relational Operator2/1, [Sat_state]
  Constant2/1 -> Relational Operator2/2
  Sign1/1 -> Relational Operator4/2, Relational Operator3/2
  Constant3/1 -> Relational Operator3/1
  Constant4/1 -> Relational Operator4/1
  Relational Operator2/1 -> Logical Operator1/2
  Relational Operator4/1 -> Logical Operator1/1
  Relational Operator3/1 -> Logical Operator2/2
  Relational Operator1/1 -> Logical Operator2/1
  Logical Operator1/1 -> Logical Operator/1
  Logical Operator2/1 -> Logical Operator/2
  Constant/1 -> Switch1/3
  Logical Operator3/1 -> Switch1/2
  Logical Operator/1 -> Logical Operator3/2
  Constant5/1 -> Relational Operator5/2
  [Sat_state] -> Relational Operator5/1
  Relational Operator5/1 -> Logical Operator3/1

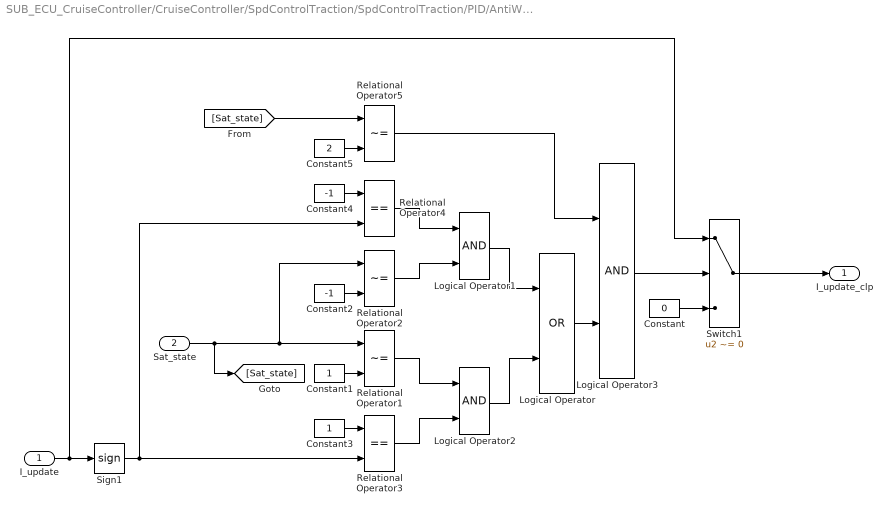
== system SUB_ECU_CruiseController/CruiseController/SpdControlTraction/SpdControlTraction/PID/AntiWindup ==
  I_update : Inport
  Sat_state : Inport  Port=2
  Constant : Constant  Value=0
  Constant1 : Constant
  Constant2 : Constant  Value=-1
  Constant3 : Constant
  Constant4 : Constant  Value=-1
  Constant5 : Constant  Value=2
  Logical Operator : Logic  Operator=OR  AllPortsSameDT=off  OutDataTypeStr=boolean
  Logical Operator1 : Logic  AllPortsSameDT=off  OutDataTypeStr=boolean
  Logical Operator2 : Logic  AllPortsSameDT=off  OutDataTypeStr=boolean
  Logical Operator3 : Logic  AllPortsSameDT=off  OutDataTypeStr=boolean
  Relational Operator1 : RelationalOperator  Operator=~=  OutDataTypeStr=boolean  RndMeth=Nearest
  Relational Operator2 : RelationalOperator  Operator=~=  OutDataTypeStr=boolean  RndMeth=Nearest
  Relational Operator3 : RelationalOperator  Operator===  OutDataTypeStr=boolean  RndMeth=Nearest
  Relational Operator4 : RelationalOperator  Operator===  OutDataTypeStr=boolean  RndMeth=Nearest
  Relational Operator5 : RelationalOperator  Operator=~=  OutDataTypeStr=boolean  RndMeth=Nearest
  Sign1 : Signum
  Switch1 : Switch  Criteria=u2 ~= 0
  I_update_clp : Outport
  wires:
  Relational Operator5/1 -> Logical Operator3/1
  [Sat_state] -> Relational Operator5/1
  Constant5/1 -> Relational Operator5/2
  Logical Operator/1 -> Logical Operator3/2
  Logical Operator3/1 -> Switch1/2
  Constant/1 -> Switch1/3
  Logical Operator2/1 -> Logical Operator/2
  Logical Operator1/1 -> Logical Operator/1
  Relational Operator1/1 -> Logical Operator2/1
  Relational Operator3/1 -> Logical Operator2/2
  Relational Operator4/1 -> Logical Operator1/1
  Relational Operator2/1 -> Logical Operator1/2
  Constant4/1 -> Relational Operator4/1
  Constant3/1 -> Relational Operator3/1
  Sign1/1 -> Relational Operator3/2, Relational Operator4/2
  Constant2/1 -> Relational Operator2/2
  Sat_state/1 -> [Sat_state], Relational Operator2/1, Relational Operator1/1
  Constant1/1 -> Relational Operator1/2
  I_update/1 -> Switch1/1, Sign1/1
  Switch1/1 -> I_update_clp/1
